simulink library "ammclib_bam_s32k11x"  (Simulink 9.0)
settings: Solver=ode45  StartTime=0.0  StopTime=10.0  RelTol=1e-3
undefined symbols (not defined in the file): f16A1, f16A2, f16B0, f16B1, f16B2, f16C1, f16CC1, f16CC1sc, f16CC1sc_D, f16CC1sc_Q, f16CC1scD, f16CC1scQ, f16CC2, f16CC2sc, f16CC2sc_D, f16CC2sc_Q, f16CC2scD, f16CC2scQ, f16DerivGain, f16EGain, f16FiltCoef, f16HystOff, f16HystOn, f16IGain, f16IntegGain, f16IntegGainFW, f16IntegGainQ, f16Kd, f16Kq, f16Limit, f16LowerLim, f16LowerLimit_D, f16LowerLimit_Q, f16ModIndex, f16OutValOff, f16OutValOn, f16PropGain, f16PropGainFW, f16PropGainQ, f16RampDown, f16RampUp, f16UGain, f16UpperLim, f16UpperLimit, f16UpperLimit_D, f16UpperLimit_Q, f16WIGain, f32A1, f32A2, f32B0, f32B1, f32B2, f32C1, f32CC1, f32CC1sc, f32CC1sc_D, f32CC1sc_Q, f32CC1scD, f32CC1scQ, f32CC2 ... (+71)
(part 3 of 7)

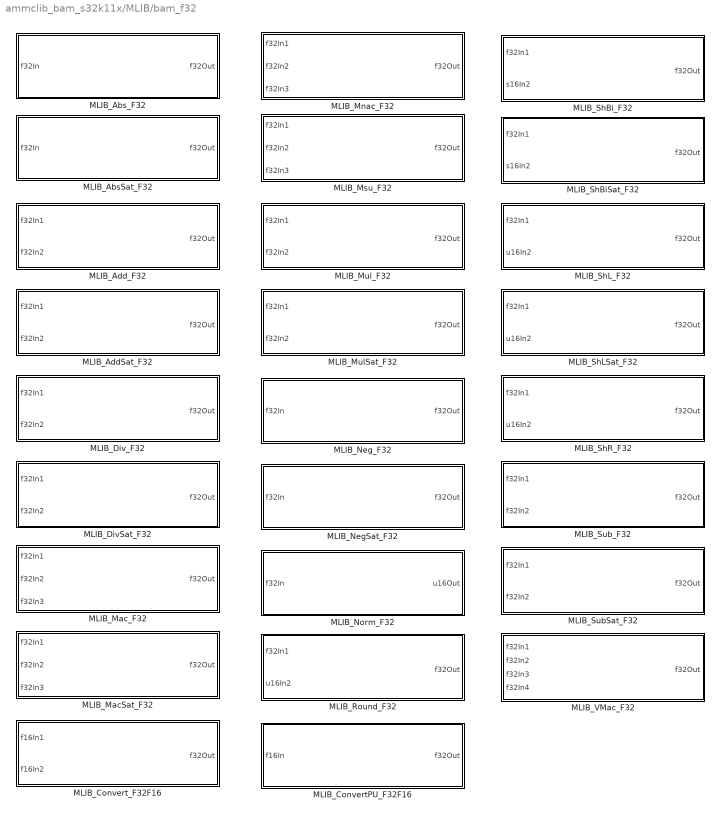
== system ammclib_bam_s32k11x/MLIB/bam_f32 ==
  MLIB_AbsSat_F32 : Subsystem  mask(MLIB_AbsSat_F32){}
      mask help: Bit accurate model for absolute value of input value. The output is saturated if necessary. All parameters as well as input and output are 32bit integers.
      mask init:
      | pos = get_param(gcb, 'Position');width = pos(3) - pos(1); height = pos(4) - pos(2);tX=width/2;tY=height*0.9;
      mask Help: web(fullfile(mbd_s32k_mc_block_help('s32k11x'), 'S32K11XMCLUG.pdf'), '-browser')
      mask Display: color('black');port_label('input',1,'f32In');port_label('output',1,'f32Out');color('black');disp('MLIB_AbsSat_F32');color('blue');text(tX,tY, 'BAM', 'horizontalAlignment', 'center');
  MLIB_Abs_F32 : Subsystem  mask(MLIB_Abs_F32){}
      mask help: Bit accurate model for absolute value of input value. All parameters as well as input and output are 32bit integers.
      mask init:
      | pos = get_param(gcb, 'Position');width = pos(3) - pos(1); height = pos(4) - pos(2);tX=width/2;tY=height*0.9;
      mask Help: web(fullfile(mbd_s32k_mc_block_help('s32k11x'), 'S32K11XMCLUG.pdf'), '-browser')
      mask Display: color('black');port_label('input',1,'f32In');port_label('output',1,'f32Out');color('black');disp('MLIB_Abs_F32');color('blue');text(tX,tY, 'BAM', 'horizontalAlignment', 'center');
  MLIB_AddSat_F32 : Subsystem  mask(MLIB_AddSat_F32){}
      mask help: Bit accurate model of saturated sum of two input values. All parameters as well as input and output are 32bit integers.
      mask init:
      | pos = get_param(gcb, 'Position');width = pos(3) - pos(1); height = pos(4) - pos(2);tX=width/2;tY=height*0.9;
      mask Help: web(fullfile(mbd_s32k_mc_block_help('s32k11x'), 'S32K11XMCLUG.pdf'), '-browser')
      mask Display: color('black');port_label('input',1,'f32In1');port_label('input',2,'f32In2');port_label('output',1,'f32Out');color('black');disp('MLIB_AddSat_F32');color('blue');text(tX,tY, 'BAM', 'horizontalAlignment', 'center');
  MLIB_Add_F32 : Subsystem  mask(MLIB_Add_F32){}
      mask help: Bit accurate model of sum of two input values. All parameters as well as input and output are 32bit integers.
      mask init:
      | pos = get_param(gcb, 'Position');width = pos(3) - pos(1); height = pos(4) - pos(2);tX=width/2;tY=height*0.9;
      mask Help: web(fullfile(mbd_s32k_mc_block_help('s32k11x'), 'S32K11XMCLUG.pdf'), '-browser')
      mask Display: color('black');port_label('input',1,'f32In1');port_label('input',2,'f32In2');port_label('output',1,'f32Out');color('black');disp('MLIB_Add_F32');color('blue');text(tX,tY, 'BAM', 'horizontalAlignment', 'center');
  MLIB_ConvertPU_F32F16 : Subsystem  mask(MLIB_ConvertPU_F32){}
      mask help: Bit accurate model for conversion value of input value. Input parameter is considered as 16-bit integer and output value is considered as 32-bit integer value.
      mask init:
      | pos = get_param(gcb, 'Position');width = pos(3) - pos(1); height = pos(4) - pos(2);tX=width/2;tY=height*0.9;
      mask Help: web(fullfile(mbd_s32k_mc_block_help('s32k11x'), 'S32K11XMCLUG.pdf'), '-browser')
      mask Display: color('black');port_label('input',1,'f16In');port_label('output',1,'f32Out');color('black');disp('MLIB_ConvertPU_F32F16');color('blue');text(tX,tY, 'BAM', 'horizontalAlignment', 'center');
  MLIB_Convert_F32F16 : Subsystem  mask(MLIB_Convert_F32F16){}
      mask help: Bit accurate model for conversion value of input value. Input parameter is considered as 16-bit integer and output value is considered as 32-bit integer value.
      mask init:
      | pos = get_param(gcb, 'Position');width = pos(3) - pos(1); height = pos(4) - pos(2);tX=width/2;tY=height*0.9;
      mask Help: web(fullfile(mbd_s32k_mc_block_help('s32k11x'), 'S32K11XMCLUG.pdf'), '-browser')
      mask Display: color('black');port_label('input',1,'f16In1');port_label('input',2,'f16In2');port_label('output',1,'f32Out');color('black');disp('MLIB_Convert_F32F16');color('blue');text(tX,tY, 'BAM', 'horizontalAlignment', 'center');
  MLIB_DivSat_F32 : Subsystem  mask(MLIB_DivSat_F32){}
      mask help: Bit accurate model of multiplication of two input values. All parameters as well as input and output are 32bit integers.
      mask init:
      | pos = get_param(gcb, 'Position');width = pos(3) - pos(1); height = pos(4) - pos(2);tX=width/2;tY=height*0.9;
      mask Help: web(fullfile(mbd_s32k_mc_block_help('s32k11x'), 'S32K11XMCLUG.pdf'), '-browser')
      mask Display: color('black');port_label('input',1,'f32In1');port_label('input',2,'f32In2');port_label('output',1,'f32Out');color('black');disp('MLIB_DivSat_F32');color('blue');text(tX,tY, 'BAM', 'horizontalAlignment', 'center');
  MLIB_Div_F32 : Subsystem  mask(MLIB_Div_F32){}
      mask help: Bit accurate model of multiplication of two input values. All parameters as well as input and output are 32bit integers.
      mask init:
      | pos = get_param(gcb, 'Position');width = pos(3) - pos(1); height = pos(4) - pos(2);tX=width/2;tY=height*0.9;
      mask Help: web(fullfile(mbd_s32k_mc_block_help('s32k11x'), 'S32K11XMCLUG.pdf'), '-browser')
      mask Display: color('black');port_label('input',1,'f32In1');port_label('input',2,'f32In2');port_label('output',1,'f32Out');color('black');disp('MLIB_Div_F32');color('blue');text(tX,tY, 'BAM', 'horizontalAlignment', 'center');
  MLIB_MacSat_F32 : Subsystem  mask(MLIB_MacSat_F32){}
      mask help: Bit accurate model of saturated multiply-accumulate of input values, saturated if necessary. All parameters as well as input and output are 32bit integers.
      mask init:
      | pos = get_param(gcb, 'Position');width = pos(3) - pos(1); height = pos(4) - pos(2);tX=width/2;tY=height*0.9;
      mask Help: web(fullfile(mbd_s32k_mc_block_help('s32k11x'), 'S32K11XMCLUG.pdf'), '-browser')
      mask Display: color('black');port_label('input',1,'f32In1');port_label('input',2,'f32In2');port_label('input',3,'f32In3');port_label('output',1,'f32Out');color('black');disp('MLIB_MacSat_F32');color('blue');text(tX,tY, 'BAM', 'horizontalAlignment', 'center');
  MLIB_Mac_F32 : Subsystem  mask(MLIB_Mac_F32){}
      mask help: Bit accurate model of multiply accumulate function. All parameters as well as input and output are 32bit integers.
      mask init:
      | pos = get_param(gcb, 'Position');width = pos(3) - pos(1); height = pos(4) - pos(2);tX=width/2;tY=height*0.9;
      mask Help: web(fullfile(mbd_s32k_mc_block_help('s32k11x'), 'S32K11XMCLUG.pdf'), '-browser')
      mask Display: color('black');port_label('input',1,'f32In1');port_label('input',2,'f32In2');port_label('input',3,'f32In3');port_label('output',1,'f32Out');color('black');disp('MLIB_Mac_F32');color('blue');text(tX,tY, 'BAM', 'horizontalAlignment', 'center');
  MLIB_Mnac_F32 : Subsystem  mask(MLIB_Mnac_F32){}
      mask help: Bit accurate model of multiply-negative-accumulate function. All parameters as well as input and output are 32bit integers.
      mask init:
      | pos = get_param(gcb, 'Position');width = pos(3) - pos(1); height = pos(4) - pos(2);tX=width/2;tY=height*0.9;
      mask Help: web(fullfile(mbd_s32k_mc_block_help('s32k11x'), 'S32K11XMCLUG.pdf'), '-browser')
      mask Display: color('black');port_label('input',1,'f32In1');port_label('input',2,'f32In2');port_label('input',3,'f32In3');port_label('output',1,'f32Out');color('black');disp('MLIB_Mnac_F32');color('blue');text(tX,tY, 'BAM', 'horizontalAlignment', 'center');
  MLIB_Msu_F32 : Subsystem  mask(MLIB_Msu_F32){}
      mask help: Bit accurate model of multiply-subtract-from function. All parameters as well as input and output are 32bit integers.
      mask init:
      | pos = get_param(gcb, 'Position');width = pos(3) - pos(1); height = pos(4) - pos(2);tX=width/2;tY=height*0.9;
      mask Help: web(fullfile(mbd_s32k_mc_block_help('s32k11x'), 'S32K11XMCLUG.pdf'), '-browser')
      mask Display: color('black');port_label('input',1,'f32In1');port_label('input',2,'f32In2');port_label('input',3,'f32In3');port_label('output',1,'f32Out');color('black');disp('MLIB_Msu_F32');color('blue');text(tX,tY, 'BAM', 'horizontalAlignment', 'center');
  MLIB_MulSat_F32 : Subsystem  mask(MLIB_MulSat_F32){}
      mask help: Bit accurate model of saturated multiplication of two input values. All parameters as well as input and output are 32bit integers.
      mask init:
      | pos = get_param(gcb, 'Position');width = pos(3) - pos(1); height = pos(4) - pos(2);tX=width/2;tY=height*0.9;
      mask Help: web(fullfile(mbd_s32k_mc_block_help('s32k11x'), 'S32K11XMCLUG.pdf'), '-browser')
      mask Display: color('black');port_label('input',1,'f32In1');port_label('input',2,'f32In2');port_label('output',1,'f32Out');color('black');disp('MLIB_MulSat_F32');color('blue');text(tX,tY, 'BAM', 'horizontalAlignment', 'center');
  MLIB_Mul_F32 : Subsystem  mask(MLIB_Mul_F32){}
      mask help: Bit accurate model of multiplication of two input values. All parameters as well as input and output are 32bit integers.
      mask init:
      | pos = get_param(gcb, 'Position');width = pos(3) - pos(1); height = pos(4) - pos(2);tX=width/2;tY=height*0.9;
      mask Help: web(fullfile(mbd_s32k_mc_block_help('s32k11x'), 'S32K11XMCLUG.pdf'), '-browser')
      mask Display: color('black');port_label('input',1,'f32In1');port_label('input',2,'f32In2');port_label('output',1,'f32Out');color('black');disp('MLIB_Mul_F32');color('blue');text(tX,tY, 'BAM', 'horizontalAlignment', 'center');
  MLIB_NegSat_F32 : Subsystem  mask(MLIB_NegSat_F32){}
      mask help: Bit accurate model for negative value of input value. The output is saturated if necessary. All parameters as well as input and output are 32bit integers.
      mask init:
      | pos = get_param(gcb, 'Position');width = pos(3) - pos(1); height = pos(4) - pos(2);tX=width/2;tY=height*0.9;
      mask Help: web(fullfile(mbd_s32k_mc_block_help('s32k11x'), 'S32K11XMCLUG.pdf'), '-browser')
      mask Display: color('black');port_label('input',1,'f32In');port_label('output',1,'f32Out');color('black');disp('MLIB_NegSat_F32');color('blue');text(tX,tY, 'BAM', 'horizontalAlignment', 'center');
  MLIB_Neg_F32 : Subsystem  mask(MLIB_Neg_F32){}
      mask help: Bit accurate model for negative value of input value. All parameters as well as input and output are 32bit integers.
      mask init:
      | pos = get_param(gcb, 'Position');width = pos(3) - pos(1); height = pos(4) - pos(2);tX=width/2;tY=height*0.9;
      mask Help: web(fullfile(mbd_s32k_mc_block_help('s32k11x'), 'S32K11XMCLUG.pdf'), '-browser')
      mask Display: color('black');port_label('input',1,'f32In');port_label('output',1,'f32Out');color('black');disp('MLIB_Neg_F32');color('blue');text(tX,tY, 'BAM', 'horizontalAlignment', 'center');
  MLIB_Norm_F32 : Subsystem  mask(MLIB_Norm_F32){}
      mask help: Bit accurate model of the normalization function. The function counts the number of left shift needed for normalization of the input fractional value.
      mask init:
      | pos = get_param(gcb, 'Position');width = pos(3) - pos(1); height = pos(4) - pos(2);tX=width/2;tY=height*0.9;
      mask Help: web(fullfile(mbd_s32k_mc_block_help('s32k11x'), 'S32K11XMCLUG.pdf'), '-browser')
      mask Display: color('black');port_label('input',1,'f32In');port_label('output',1,'u16Out');color('black');disp('MLIB_Norm_F32');color('blue');text(tX,tY, 'BAM', 'horizontalAlignment', 'center');
  MLIB_Round_F32 : Subsystem  mask(MLIB_Round_F32){}
      mask help: Bit accurate model of the fuction rounds the first input value for number of digits defined by second parameter and saturate automaticaly. All parameters as well as input and output are 32bit integers.
      mask init:
      | pos = get_param(gcb, 'Position');width = pos(3) - pos(1); height = pos(4) - pos(2);tX=width/2;tY=height*0.9;
      mask Help: web(fullfile(mbd_s32k_mc_block_help('s32k11x'), 'S32K11XMCLUG.pdf'), '-browser')
      mask Display: color('black');port_label('input',1,'f32In1');port_label('input',2,'u16In2');port_label('output',1,'f32Out');color('black');disp('MLIB_Round_F32');color('blue');text(tX,tY, 'BAM', 'horizontalAlignment', 'center');
  MLIB_ShBiSat_F32 : Subsystem  mask(MLIB_ShBiSat_F32){}
      mask help: Bit accurate model of the fuction shifts the first parameter to left or right by number defined by second parameter and saturate if necessary. If the sign of second parameter is negative, shift to right. All parameters as well as input and output are 32bit integers.
      mask init:
      | pos = get_param(gcb, 'Position');width = pos(3) - pos(1); height = pos(4) - pos(2);tX=width/2;tY=height*0.9;
      mask Help: web(fullfile(mbd_s32k_mc_block_help('s32k11x'), 'S32K11XMCLUG.pdf'), '-browser')
      mask Display: color('black');port_label('input',1,'f32In1');port_label('input',2,'s16In2');port_label('output',1,'f32Out');color('black');disp('MLIB_ShBiSat_F32');color('blue');text(tX,tY, 'BAM', 'horizontalAlignment', 'center');
  MLIB_ShBi_F32 : Subsystem  mask(MLIB_ShBi_F32){}
      mask help: Bit accurate model of the fuction shifts the first parameter to left or right by number defined by second parameter. If the sign of second parameter is negative, shift to right. All parameters as well as input and output are 16bit integers.
      mask init:
      | pos = get_param(gcb, 'Position');width = pos(3) - pos(1); height = pos(4) - pos(2);tX=width/2;tY=height*0.9;
      mask Help: web(fullfile(mbd_s32k_mc_block_help('s32k11x'), 'S32K11XMCLUG.pdf'), '-browser')
      mask Display: color('black');port_label('input',1,'f32In1');port_label('input',2,'s16In2');port_label('output',1,'f32Out');color('black');disp('MLIB_ShBi_F32');color('blue');text(tX,tY, 'BAM', 'horizontalAlignment', 'center');
  MLIB_ShLSat_F32 : Subsystem  mask(MLIB_ShLSat_F32){}
      mask help: Bit accurate model of the fuction shifts the first parameter to left by number defined by second parameter and saturate if necessary. All parameters as well as input and output are 32bit integers.
      mask init:
      | pos = get_param(gcb, 'Position');width = pos(3) - pos(1); height = pos(4) - pos(2);tX=width/2;tY=height*0.9;
      mask Help: web(fullfile(mbd_s32k_mc_block_help('s32k11x'), 'S32K11XMCLUG.pdf'), '-browser')
      mask Display: color('black');port_label('input',1,'f32In1');port_label('input',2,'u16In2');port_label('output',1,'f32Out');color('black');disp('MLIB_ShLSat_F32');color('blue');text(tX,tY, 'BAM', 'horizontalAlignment', 'center');
  MLIB_ShL_F32 : Subsystem  mask(MLIB_ShL_F32){}
      mask help: Bit accurate model of the fuction shifts the first parameter to left by number defined by second parameter. All parameters as well as input and output are 32bit integers.
      mask init:
      | pos = get_param(gcb, 'Position');width = pos(3) - pos(1); height = pos(4) - pos(2);tX=width/2;tY=height*0.9;
      mask Help: web(fullfile(mbd_s32k_mc_block_help('s32k11x'), 'S32K11XMCLUG.pdf'), '-browser')
      mask Display: color('black');port_label('input',1,'f32In1');port_label('input',2,'u16In2');port_label('output',1,'f32Out');color('black');disp('MLIB_ShL_F32');color('blue');text(tX,tY, 'BAM', 'horizontalAlignment', 'center');
  MLIB_ShR_F32 : Subsystem  mask(MLIB_ShR_F32){}
      mask help: Bit accurate model of the fuction shifts the first parameter to right by number defined by second parameter. All parameters as well as input and output are 32bit integers.
      mask init:
      | pos = get_param(gcb, 'Position');width = pos(3) - pos(1); height = pos(4) - pos(2);tX=width/2;tY=height*0.9;
      mask Help: web(fullfile(mbd_s32k_mc_block_help('s32k11x'), 'S32K11XMCLUG.pdf'), '-browser')
      mask Display: color('black');port_label('input',1,'f32In1');port_label('input',2,'u16In2');port_label('output',1,'f32Out');color('black');disp('MLIB_ShR_F32');color('blue');text(tX,tY, 'BAM', 'horizontalAlignment', 'center');
  MLIB_SubSat_F32 : Subsystem  mask(MLIB_SubSat_F32){}
      mask help: Bit accurate model of saturated subtraction of two input values. All parameters as well as input and output are 32bit integers.
      mask init:
      | pos = get_param(gcb, 'Position');width = pos(3) - pos(1); height = pos(4) - pos(2);tX=width/2;tY=height*0.9;
      mask Help: web(fullfile(mbd_s32k_mc_block_help('s32k11x'), 'S32K11XMCLUG.pdf'), '-browser')
      mask Display: color('black');port_label('input',1,'f32In1');port_label('input',2,'f32In2');port_label('output',1,'f32Out');color('black');disp('MLIB_SubSat_F32');color('blue');text(tX,tY, 'BAM', 'horizontalAlignment', 'center');
  MLIB_Sub_F32 : Subsystem  mask(MLIB_Sub_F32){}
      mask help: Bit accurate model of subtract of two input values. All parameters as well as input and output are 32bit integers.
      mask init:
      | pos = get_param(gcb, 'Position');width = pos(3) - pos(1); height = pos(4) - pos(2);tX=width/2;tY=height*0.9;
      mask Help: web(fullfile(mbd_s32k_mc_block_help('s32k11x'), 'S32K11XMCLUG.pdf'), '-browser')
      mask Display: color('black');port_label('input',1,'f32In1');port_label('input',2,'f32In2');port_label('output',1,'f32Out');color('black');disp('MLIB_Sub_F32');color('blue');text(tX,tY, 'BAM', 'horizontalAlignment', 'center');
  MLIB_VMac_F32 : Subsystem  mask(MLIB_VMac_F32){}
      mask help: Bit accurate model of vector multiply accumulate function. All parameters as well as input and output are 32-bit integers.
      mask init:
      | pos = get_param(gcb, 'Position');width = pos(3) - pos(1); height = pos(4) - pos(2);tX=width/2;tY=height*0.9;
      mask Help: web(fullfile(mbd_s32k_mc_block_help('s32k11x'), 'S32K11XMCLUG.pdf'), '-browser')
      mask Display: color('black');port_label('input',1,'f32In1');port_label('input',2,'f32In2');port_label('input',3,'f32In3');port_label('input',4,'f32In4');port_label('output',1,'f32Out');color('black');disp('MLIB_VMac_F32');color('blue');text(tX,tY, 'BAM', 'horizontalAlignment', 'center');

== system ammclib_bam_s32k11x/MLIB/bam_f32f16f16 ==
  MLIB_MacSat_F32F16F16 : Subsystem  mask(MLIB_MacSat_F32F16F16){}
      mask help: Bit accurate model of saturated multiply-accumulate of input values, saturated if necessary. All input parameters are 16bit integers, output value is 32-bit integer.
      mask init:
      | pos = get_param(gcb, 'Position');width = pos(3) - pos(1); height = pos(4) - pos(2);tX=width/2;tY=height*0.9;
      mask Help: web(fullfile(mbd_s32k_mc_block_help('s32k11x'), 'S32K11XMCLUG.pdf'), '-browser')
      mask Display: color('black');port_label('input',1,'f32In1');port_label('input',2,'f16In2');port_label('input',3,'f16In3');port_label('output',1,'f32Out');color('black');disp('MLIB_MacSat_F32F16F16');color('blue');text(tX,tY, 'BAM', 'horizontalAlignment', 'center');
  MLIB_Mac_F32F16F16 : Subsystem  mask(MLIB_Mac_F32F16F16){}
      mask help: Bit accurate model of multiply accumulate function. First input parameters as well as output are 32bit integers. Second and third parameters are 16-bit integers.
      mask init:
      | pos = get_param(gcb, 'Position');width = pos(3) - pos(1); height = pos(4) - pos(2);tX=width/2;tY=height*0.9;
      mask Help: web(fullfile(mbd_s32k_mc_block_help('s32k11x'), 'S32K11XMCLUG.pdf'), '-browser')
      mask Display: color('black');port_label('input',1,'f32In1');port_label('input',2,'f16In2');port_label('input',3,'f16In3');port_label('output',1,'f32Out');color('black');disp('MLIB_Mac_F32F16F16');color('blue');text(tX,tY, 'BAM', 'horizontalAlignment', 'center');
  MLIB_Mnac_F32F16F16 : Subsystem  mask(MLIB_Mnac_F32F16F16){}
      mask help: Bit accurate model of multiply-negative-accumulate function. First input parameters as well as output are 32bit integers. Second and third parameters are 16-bit integers.
      mask init:
      | pos = get_param(gcb, 'Position');width = pos(3) - pos(1); height = pos(4) - pos(2);tX=width/2;tY=height*0.9;
      mask Help: web(fullfile(mbd_s32k_mc_block_help('s32k11x'), 'S32K11XMCLUG.pdf'), '-browser')
      mask Display: color('black');port_label('input',1,'f32In1');port_label('input',2,'f16In2');port_label('input',3,'f16In3');port_label('output',1,'f32Out');color('black');disp('MLIB_Mnac_F32F16F16');color('blue');text(tX,tY, 'BAM', 'horizontalAlignment', 'center');
  MLIB_Msu_F32F16F16 : Subsystem  mask(MLIB_Msu_F32F16F16){}
      mask help: Bit accurate model of multiply-subtract-from function. First input parameter as well as output are 32bit integers. Second and third parameters are 16-bit integers.
      mask init:
      | pos = get_param(gcb, 'Position');width = pos(3) - pos(1); height = pos(4) - pos(2);tX=width/2;tY=height*0.9;
      mask Help: web(fullfile(mbd_s32k_mc_block_help('s32k11x'), 'S32K11XMCLUG.pdf'), '-browser')
      mask Display: color('black');port_label('input',1,'f32In1');port_label('input',2,'f16In2');port_label('input',3,'f16In3');port_label('output',1,'f32Out');color('black');disp('MLIB_Msu_F32F16F16');color('blue');text(tX,tY, 'BAM', 'horizontalAlignment', 'center');
  MLIB_MulSat_F32F16F16 : Subsystem  mask(MLIB_MulSat_F32F16F16){}
      mask help: Bit accurate model of saturated multiplication of two input values. All input parameters are 16bit integers, output value is 32-bit integer.
      mask init:
      | pos = get_param(gcb, 'Position');width = pos(3) - pos(1); height = pos(4) - pos(2);tX=width/2;tY=height*0.9;
      mask Help: web(fullfile(mbd_s32k_mc_block_help('s32k11x'), 'S32K11XMCLUG.pdf'), '-browser')
      mask Display: color('black');port_label('input',1,'f16In1');port_label('input',2,'f16In2');port_label('output',1,'f32Out');color('black');disp('MLIB_MulSat_F32F16F16');color('blue');text(tX,tY, 'BAM', 'horizontalAlignment', 'center');
  MLIB_Mul_F32F16F16 : Subsystem  mask(MLIB_Mul_F32F16F16){}
      mask help: Bit accurate model of multiplication of two input values. Both input parameters are 16bit integers and output value is 32-bit integer.
      mask init:
      | pos = get_param(gcb, 'Position');width = pos(3) - pos(1); height = pos(4) - pos(2);tX=width/2;tY=height*0.9;
      mask Help: web(fullfile(mbd_s32k_mc_block_help('s32k11x'), 'S32K11XMCLUG.pdf'), '-browser')
      mask Display: color('black');port_label('input',1,'f16In1');port_label('input',2,'f16In2');port_label('output',1,'f32Out');color('black');disp('MLIB_Mul_F32F16F16');color('blue');text(tX,tY, 'BAM', 'horizontalAlignment', 'center');
  MLIB_VMac_F32F16F16 : Subsystem  mask(MLIB_VMac_F32F16F16){}
      mask help: Bit accurate model of vector multiply accumulate function. The input parameters are 16-bit integers, the output value is 32-bit integer.
      mask init:
      | pos = get_param(gcb, 'Position');width = pos(3) - pos(1); height = pos(4) - pos(2);tX=width/2;tY=height*0.9;
      mask Help: web(fullfile(mbd_s32k_mc_block_help('s32k11x'), 'S32K11XMCLUG.pdf'), '-browser')
      mask Display: color('black');port_label('input',1,'f16In1');port_label('input',2,'f16In2');port_label('input',3,'f16In3');port_label('input',4,'f16In4');port_label('output',1,'f32Out');color('black');disp('MLIB_VMac_F32F16F16');color('blue');text(tX,tY, 'BAM', 'horizontalAlignment', 'center');

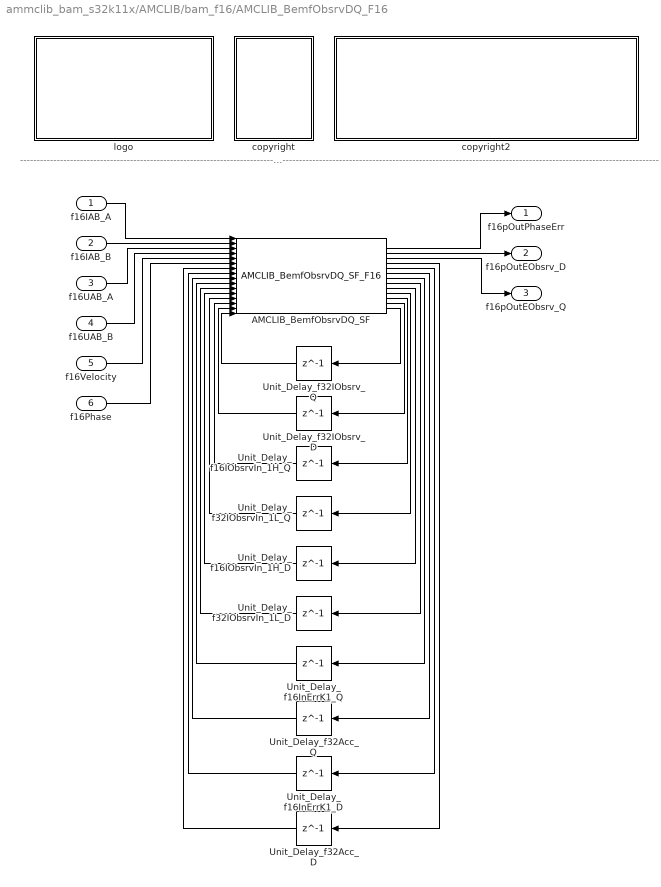
== system ammclib_bam_s32k11x/AMCLIB/bam_f16/AMCLIB_BemfObsrvDQ_F16 ==
  note: ---------------------------------------------------------------------------------------------------------------------------------------------------------------------------------------------------
  f16IAB_A : Inport
  f16IAB_B : Inport  Port=2
  f16UAB_A : Inport  Port=3
  f16UAB_B : Inport  Port=4
  f16Velocity : Inport  Port=5
  f16Phase : Inport  Port=6
  AMCLIB_BemfObsrvDQ_SF : S-Function  FunctionName=AMCLIB_BemfObsrvDQ_SF_F16  Parameters=f16IGain,f16UGain,f16WIGain,f16EGain,s16Shift,f16CC1sc_D,f16CC1sc_Q,f16CC2sc_D,f16CC2sc_Q,f16UpperLimit_D,f16UpperLimit_Q,f16LowerLimit_D,f16LowerLimit_Q,u16NShift  SFunctionDeploymentMode=off  EnableBusSupport=off
  Unit_Delay_f16IObsrvIn_1H_D : Delay  DelayLength=1  InitialCondition=0
  Unit_Delay_f16IObsrvIn_1H_Q : Delay  DelayLength=1  InitialCondition=0
  Unit_Delay_f16InErrK1_D : Delay  DelayLength=1  InitialCondition=0
  Unit_Delay_f16InErrK1_Q : Delay  DelayLength=1  InitialCondition=0
  Unit_Delay_f32Acc_D : Delay  DelayLength=1  InitialCondition=0
  Unit_Delay_f32Acc_Q : Delay  DelayLength=1  InitialCondition=0
  Unit_Delay_f32IObsrvIn_1L_D : Delay  DelayLength=1  InitialCondition=0
  Unit_Delay_f32IObsrvIn_1L_Q : Delay  DelayLength=1  InitialCondition=0
  Unit_Delay_f32IObsrv_D : Delay  DelayLength=1  InitialCondition=0
  Unit_Delay_f32IObsrv_Q : Delay  DelayLength=1  InitialCondition=0
  copyright : Subsystem
      mask Display: text(10,90,'FILE:');text(10,75,'DESRIPTION:');text(10,60,'COPYRIGHT:');text(10,45,'VERSION:');text(10,30,'DATE:')
  copyright2 : Subsystem
      mask Display: text(10,90,'AMCLIB_BemfObsrvDQ_BAM_F16.mdl');text(10,75,'PMSM back-EMF observer DQ.');text(10,60,'NXP');text(10,45,'1.0');text(10,30,'26-Oct-2016');
  logo : Subsystem
      mask Display: image(imread('logo.jpg'))
  f16pOutPhaseErr : Outport
  f16pOutEObsrv_D : Outport  Port=2
  f16pOutEObsrv_Q : Outport  Port=3
  wires:
  f16IAB_A/1 -> AMCLIB_BemfObsrvDQ_SF/1
  f16IAB_B/1 -> AMCLIB_BemfObsrvDQ_SF/2
  f16UAB_A/1 -> AMCLIB_BemfObsrvDQ_SF/3
  f16UAB_B/1 -> AMCLIB_BemfObsrvDQ_SF/4
  f16Velocity/1 -> AMCLIB_BemfObsrvDQ_SF/5
  f16Phase/1 -> AMCLIB_BemfObsrvDQ_SF/6
  AMCLIB_BemfObsrvDQ_SF/1 -> f16pOutPhaseErr/1
  AMCLIB_BemfObsrvDQ_SF/2 -> f16pOutEObsrv_D/1
  AMCLIB_BemfObsrvDQ_SF/3 -> f16pOutEObsrv_Q/1
  Unit_Delay_f32IObsrv_Q/1 -> AMCLIB_BemfObsrvDQ_SF/16
  Unit_Delay_f32IObsrv_D/1 -> AMCLIB_BemfObsrvDQ_SF/15
  Unit_Delay_f16IObsrvIn_1H_Q/1 -> AMCLIB_BemfObsrvDQ_SF/14
  AMCLIB_BemfObsrvDQ_SF/13 -> Unit_Delay_f32IObsrv_Q/1
  AMCLIB_BemfObsrvDQ_SF/12 -> Unit_Delay_f32IObsrv_D/1
  AMCLIB_BemfObsrvDQ_SF/11 -> Unit_Delay_f16IObsrvIn_1H_Q/1
  Unit_Delay_f32IObsrvIn_1L_Q/1 -> AMCLIB_BemfObsrvDQ_SF/13
  AMCLIB_BemfObsrvDQ_SF/10 -> Unit_Delay_f32IObsrvIn_1L_Q/1
  Unit_Delay_f16IObsrvIn_1H_D/1 -> AMCLIB_BemfObsrvDQ_SF/12
  AMCLIB_BemfObsrvDQ_SF/9 -> Unit_Delay_f16IObsrvIn_1H_D/1
  Unit_Delay_f32IObsrvIn_1L_D/1 -> AMCLIB_BemfObsrvDQ_SF/11
  AMCLIB_BemfObsrvDQ_SF/8 -> Unit_Delay_f32IObsrvIn_1L_D/1
  Unit_Delay_f16InErrK1_Q/1 -> AMCLIB_BemfObsrvDQ_SF/10
  AMCLIB_BemfObsrvDQ_SF/7 -> Unit_Delay_f16InErrK1_Q/1
  Unit_Delay_f32Acc_Q/1 -> AMCLIB_BemfObsrvDQ_SF/9
  AMCLIB_BemfObsrvDQ_SF/6 -> Unit_Delay_f32Acc_Q/1
  AMCLIB_BemfObsrvDQ_SF/5 -> Unit_Delay_f16InErrK1_D/1
  Unit_Delay_f16InErrK1_D/1 -> AMCLIB_BemfObsrvDQ_SF/8
  Unit_Delay_f32Acc_D/1 -> AMCLIB_BemfObsrvDQ_SF/7
  AMCLIB_BemfObsrvDQ_SF/4 -> Unit_Delay_f32Acc_D/1

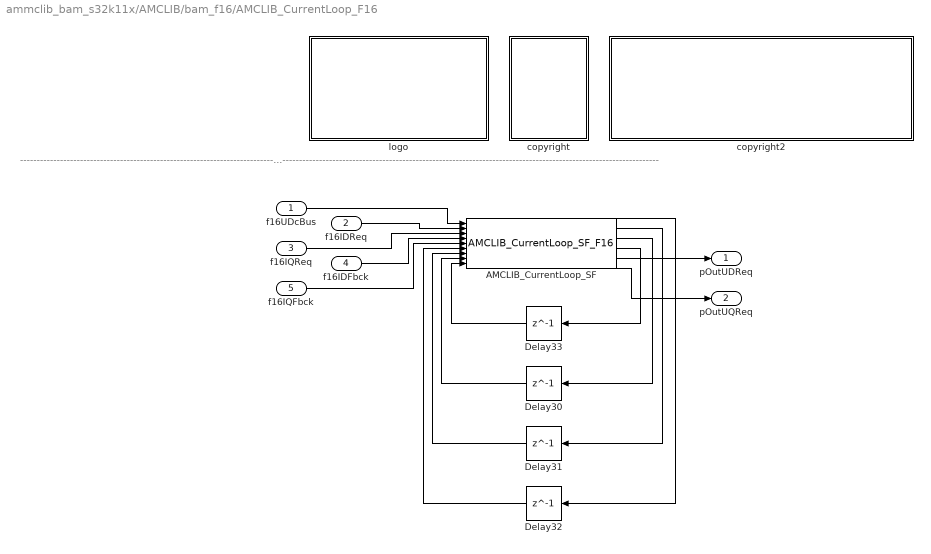
== system ammclib_bam_s32k11x/AMCLIB/bam_f16/AMCLIB_CurrentLoop_F16 ==
  note: ---------------------------------------------------------------------------------------------------------------------------------------------------------------------------------------------------
  f16UDcBus : Inport
  f16IDReq : Inport  Port=2
  f16IQReq : Inport  Port=3
  f16IDFbck : Inport  Port=4
  f16IQFbck : Inport  Port=5
  AMCLIB_CurrentLoop_SF : S-Function  FunctionName=AMCLIB_CurrentLoop_SF_F16  Parameters=f16CC1scD,f16CC2scD,u16NShiftD,f16CC1scQ,f16CC2scQ,u16NShiftQ  SFunctionDeploymentMode=off  EnableBusSupport=off
  Delay{30..33} (4 alike) : Delay  DelayLength=1  InitialCondition=0
  copyright : Subsystem
      mask Display: text(10,90,'FILE:');text(10,75,'DESRIPTION:');text(10,60,'COPYRIGHT:');text(10,45,'VERSION:');text(10,30,'DATE:')
  copyright2 : Subsystem
      mask Display: text(10,90,'AMCLIB_CurrentLoop_BAM_F16.mdl');text(10,75,'PMSM Current Loop.');text(10,60,'NXP');text(10,45,'1.0');text(10,30,'25-Oct-2017');
  logo : Subsystem
      mask Display: image(imread('logo.jpg'))
  pOutUDReq : Outport
  pOutUQReq : Outport  Port=2
  wires:
  f16UDcBus/1 -> AMCLIB_CurrentLoop_SF/1
  f16IDReq/1 -> AMCLIB_CurrentLoop_SF/2
  f16IQReq/1 -> AMCLIB_CurrentLoop_SF/3
  f16IDFbck/1 -> AMCLIB_CurrentLoop_SF/4
  f16IQFbck/1 -> AMCLIB_CurrentLoop_SF/5
  Delay32/1 -> AMCLIB_CurrentLoop_SF/6
  Delay31/1 -> AMCLIB_CurrentLoop_SF/7
  Delay30/1 -> AMCLIB_CurrentLoop_SF/8
  Delay33/1 -> AMCLIB_CurrentLoop_SF/9
  AMCLIB_CurrentLoop_SF/1 -> Delay32/1
  AMCLIB_CurrentLoop_SF/2 -> Delay31/1
  AMCLIB_CurrentLoop_SF/3 -> Delay30/1
  AMCLIB_CurrentLoop_SF/4 -> Delay33/1
  AMCLIB_CurrentLoop_SF/5 -> pOutUDReq/1
  AMCLIB_CurrentLoop_SF/6 -> pOutUQReq/1

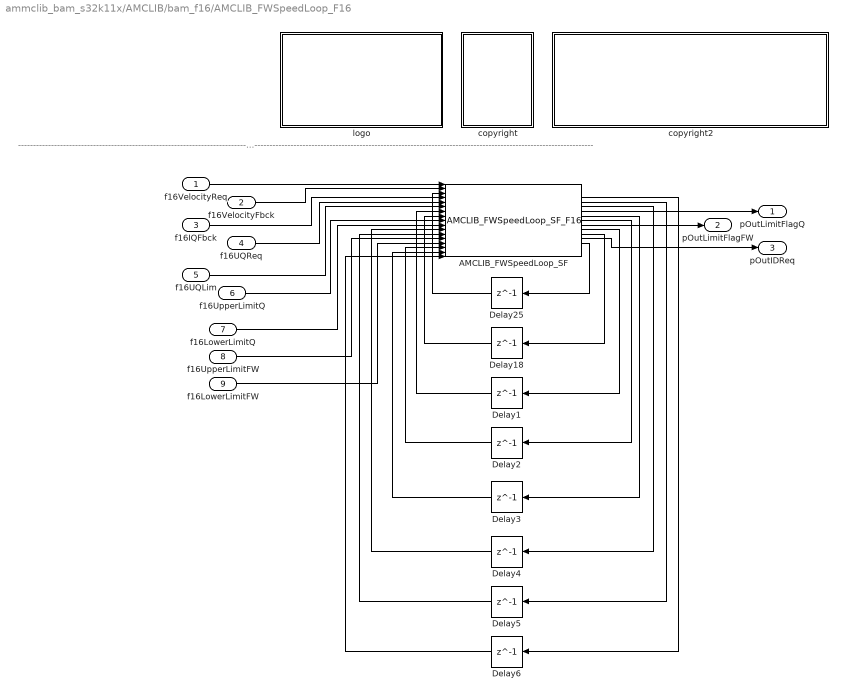
== system ammclib_bam_s32k11x/AMCLIB/bam_f16/AMCLIB_FWSpeedLoop_F16 ==
  note: ---------------------------------------------------------------------------------------------------------------------------------------------------------------------------------------------------
  f16VelocityReq : Inport
  f16VelocityFbck : Inport  Port=2
  f16IQFbck : Inport  Port=3
  f16UQReq : Inport  Port=4
  f16UQLim : Inport  Port=5
  f16UpperLimitQ : Inport  Port=6
  f16LowerLimitQ : Inport  Port=7
  f16UpperLimitFW : Inport  Port=8
  f16LowerLimitFW : Inport  Port=9
  AMCLIB_FWSpeedLoop_SF : S-Function  FunctionName=AMCLIB_FWSpeedLoop_SF_F16  Parameters=u16NSamplesW,u16NSamplesFW,f16PropGainQ,s16PropGainShiftQ,f16IntegGainQ,s16IntegGainShiftQ,f16PropGainFW,s16PropGainShiftFW,f16IntegGainFW,s16IntegGainShiftFW,f32RampUp,f32RampDown  SFunctionDeploymentMode=off  EnableBusSupport=off
  Delay{1..6,18,25} (8 alike) : Delay  DelayLength=1  InitialCondition=0
  copyright : Subsystem
      mask Display: text(10,90,'FILE:');text(10,75,'DESRIPTION:');text(10,60,'COPYRIGHT:');text(10,45,'VERSION:');text(10,30,'DATE:')
  copyright2 : Subsystem
      mask Display: text(10,90,'AMCLIB_FWSpeedLoop_BAM_F16.mdl');text(10,75,'Speed Loop with Field Weakening.');text(10,60,'NXP');text(10,45,'1.0');text(10,30,'28-Aug-2017');
  logo : Subsystem
      mask Display: image(imread('logo.jpg'))
  pOutLimitFlagQ : Outport
  pOutLimitFlagFW : Outport  Port=2
  pOutIDReq : Outport  Port=3
  wires:
  f16VelocityReq/1 -> AMCLIB_FWSpeedLoop_SF/1
  f16VelocityFbck/1 -> AMCLIB_FWSpeedLoop_SF/2
  Delay25/1 -> AMCLIB_FWSpeedLoop_SF/3
  f16IQFbck/1 -> AMCLIB_FWSpeedLoop_SF/4
  f16UQReq/1 -> AMCLIB_FWSpeedLoop_SF/5
  f16UQLim/1 -> AMCLIB_FWSpeedLoop_SF/6
  Delay1/1 -> AMCLIB_FWSpeedLoop_SF/7
  Delay18/1 -> AMCLIB_FWSpeedLoop_SF/8
  f16UpperLimitQ/1 -> AMCLIB_FWSpeedLoop_SF/9
  f16LowerLimitQ/1 -> AMCLIB_FWSpeedLoop_SF/10
  Delay4/1 -> AMCLIB_FWSpeedLoop_SF/11
  Delay5/1 -> AMCLIB_FWSpeedLoop_SF/12
  f16UpperLimitFW/1 -> AMCLIB_FWSpeedLoop_SF/13
  f16LowerLimitFW/1 -> AMCLIB_FWSpeedLoop_SF/14
  Delay2/1 -> AMCLIB_FWSpeedLoop_SF/15
  Delay3/1 -> AMCLIB_FWSpeedLoop_SF/16
  Delay6/1 -> AMCLIB_FWSpeedLoop_SF/17
  AMCLIB_FWSpeedLoop_SF/1 -> Delay6/1
  AMCLIB_FWSpeedLoop_SF/2 -> Delay5/1
  AMCLIB_FWSpeedLoop_SF/3 -> Delay4/1
  AMCLIB_FWSpeedLoop_SF/4 -> pOutLimitFlagQ/1
  AMCLIB_FWSpeedLoop_SF/5 -> Delay3/1
  AMCLIB_FWSpeedLoop_SF/6 -> Delay2/1
  AMCLIB_FWSpeedLoop_SF/7 -> pOutLimitFlagFW/1
  AMCLIB_FWSpeedLoop_SF/8 -> Delay1/1
  AMCLIB_FWSpeedLoop_SF/9 -> Delay18/1
  AMCLIB_FWSpeedLoop_SF/10 -> pOutIDReq/1
  AMCLIB_FWSpeedLoop_SF/11 -> Delay25/1

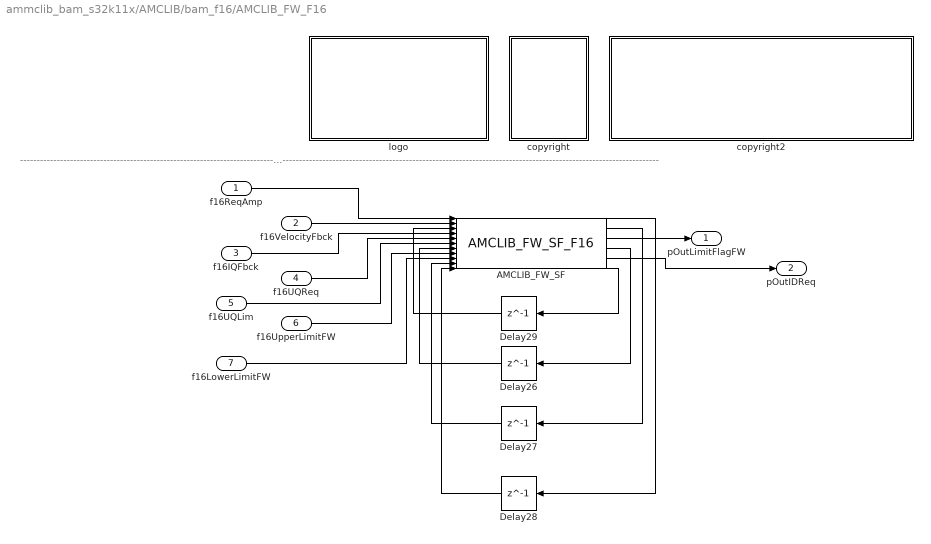
== system ammclib_bam_s32k11x/AMCLIB/bam_f16/AMCLIB_FW_F16 ==
  note: ---------------------------------------------------------------------------------------------------------------------------------------------------------------------------------------------------
  f16ReqAmp : Inport
  f16VelocityFbck : Inport  Port=2
  f16IQFbck : Inport  Port=3
  f16UQReq : Inport  Port=4
  f16UQLim : Inport  Port=5
  f16UpperLimitFW : Inport  Port=6
  f16LowerLimitFW : Inport  Port=7
  AMCLIB_FW_SF : S-Function  FunctionName=AMCLIB_FW_SF_F16  Parameters=u16NSamplesFW,f16PropGainFW,s16PropGainShiftFW,f16IntegGainFW,s16IntegGainShiftFW  SFunctionDeploymentMode=off  EnableBusSupport=off
  Delay{26..29} (4 alike) : Delay  DelayLength=1  InitialCondition=0
  copyright : Subsystem
      mask Display: text(10,90,'FILE:');text(10,75,'DESRIPTION:');text(10,60,'COPYRIGHT:');text(10,45,'VERSION:');text(10,30,'DATE:')
  copyright2 : Subsystem
      mask Display: text(10,90,'AMCLIB_FW_BAM_F16.mdl');text(10,75,'Speed Loop with Field Weakening.');text(10,60,'NXP');text(10,45,'1.0');text(10,30,'28-Aug-2017');
  logo : Subsystem
      mask Display: image(imread('logo.jpg'))
  pOutLimitFlagFW : Outport
  pOutIDReq : Outport  Port=2
  wires:
  f16ReqAmp/1 -> AMCLIB_FW_SF/1
  f16VelocityFbck/1 -> AMCLIB_FW_SF/2
  Delay29/1 -> AMCLIB_FW_SF/3
  f16IQFbck/1 -> AMCLIB_FW_SF/4
  f16UQReq/1 -> AMCLIB_FW_SF/5
  f16UQLim/1 -> AMCLIB_FW_SF/6
  Delay26/1 -> AMCLIB_FW_SF/7
  f16UpperLimitFW/1 -> AMCLIB_FW_SF/8
  f16LowerLimitFW/1 -> AMCLIB_FW_SF/9
  Delay27/1 -> AMCLIB_FW_SF/10
  Delay28/1 -> AMCLIB_FW_SF/11
  AMCLIB_FW_SF/1 -> Delay28/1
  AMCLIB_FW_SF/2 -> Delay27/1
  AMCLIB_FW_SF/3 -> pOutLimitFlagFW/1
  AMCLIB_FW_SF/4 -> Delay26/1
  AMCLIB_FW_SF/5 -> pOutIDReq/1
  AMCLIB_FW_SF/6 -> Delay29/1

== system ammclib_bam_s32k11x/AMCLIB/bam_f16/AMCLIB_SpeedLoop_F16 ==
  note: ---------------------------------------------------------------------------------------------------------------------------------------------------------------------------------------------------
  f16VelocityReq : Inport
  f16VelocityFbck : Inport  Port=2
  f16UpperLimitQ : Inport  Port=3
  f16LowerLimitQ : Inport  Port=4
  AMCLIB_SpeedLoop_SF : S-Function  FunctionName=AMCLIB_SpeedLoop_SF_F16  Parameters=u16NSamplesW,f16PropGainQ,s16PropGainShiftQ,f16IntegGainQ,s16IntegGainShiftQ,f32RampUp,f32RampDown  SFunctionDeploymentMode=off  EnableBusSupport=off
  Delay{1..3,17} (4 alike) : Delay  DelayLength=1  InitialCondition=0
  copyright : Subsystem
      mask Display: text(10,90,'FILE:');text(10,75,'DESRIPTION:');text(10,60,'COPYRIGHT:');text(10,45,'VERSION:');text(10,30,'DATE:')
  copyright2 : Subsystem
      mask Display: text(10,90,'AMCLIB_SpeedLoop_BAM_F16.mdl');text(10,75,'Speed Loop with Field Weakening.');text(10,60,'NXP');text(10,45,'1.0');text(10,30,'28-Aug-2017');
  logo : Subsystem
      mask Display: image(imread('logo.jpg'))
  pOutLimitFlagQ : Outport
  pOutIQReq : Outport  Port=2
  wires:
  f16VelocityReq/1 -> AMCLIB_SpeedLoop_SF/1
  f16VelocityFbck/1 -> AMCLIB_SpeedLoop_SF/2
  Delay17/1 -> AMCLIB_SpeedLoop_SF/3
  f16UpperLimitQ/1 -> AMCLIB_SpeedLoop_SF/4
  f16LowerLimitQ/1 -> AMCLIB_SpeedLoop_SF/5
  Delay1/1 -> AMCLIB_SpeedLoop_SF/6
  Delay2/1 -> AMCLIB_SpeedLoop_SF/7
  Delay3/1 -> AMCLIB_SpeedLoop_SF/8
  AMCLIB_SpeedLoop_SF/1 -> Delay3/1
  AMCLIB_SpeedLoop_SF/2 -> Delay2/1
  AMCLIB_SpeedLoop_SF/3 -> Delay1/1
  AMCLIB_SpeedLoop_SF/4 -> pOutLimitFlagQ/1
  AMCLIB_SpeedLoop_SF/6 -> pOutIQReq/1
  AMCLIB_SpeedLoop_SF/5 -> Delay17/1

== system ammclib_bam_s32k11x/AMCLIB/bam_f16/AMCLIB_TrackObsrv_F16 ==
  note: ---------------------------------------------------------------------------------------------------------------------------------------------------------------------------------------------------
  f16PhaseErr : Inport
  f16UpperLimit : Inport  Port=2
  f16LowerLimit : Inport  Port=3
  AMCLIB_TrackObsrv_SF : S-Function  FunctionName=AMCLIB_TrackObsrv_SF_F16  Parameters=f16CC1sc,f16CC2sc,u16NShift,f16C1,u16IntegNShift  SFunctionDeploymentMode=off  EnableBusSupport=off
  Unit_Delay_f16InErrK1 : Delay  DelayLength=1  InitialCondition=0
  Unit_Delay_f16InK1 : Delay  DelayLength=1  InitialCondition=0
  Unit_Delay_f32Acc : Delay  DelayLength=1  InitialCondition=0
  Unit_Delay_f32State : Delay  DelayLength=1  InitialCondition=0
  copyright : Subsystem
      mask Display: text(10,90,'FILE:');text(10,75,'DESRIPTION:');text(10,60,'COPYRIGHT:');text(10,45,'VERSION:');text(10,30,'DATE:')
  copyright2 : Subsystem
      mask Display: text(10,90,'AMCLIB_TrackObsrv_BAM_F16.mdl');text(10,75,'Tracking observer function.');text(10,60,'NXP');text(10,45,'1.0');text(10,30,'29-Jul-2016');
  logo : Subsystem
      mask Display: image(imread('logo.jpg'))
  f16PosEst : Outport
  f16VelocityEst : Outport  Port=2
  wires:
  AMCLIB_TrackObsrv_SF/2 -> f16VelocityEst/1
  AMCLIB_TrackObsrv_SF/1 -> f16PosEst/1
  f16LowerLimit/1 -> AMCLIB_TrackObsrv_SF/5
  f16UpperLimit/1 -> AMCLIB_TrackObsrv_SF/4
  f16PhaseErr/1 -> AMCLIB_TrackObsrv_SF/1
  Unit_Delay_f16InK1/1 -> AMCLIB_TrackObsrv_SF/7
  Unit_Delay_f32State/1 -> AMCLIB_TrackObsrv_SF/6
  Unit_Delay_f16InErrK1/1 -> AMCLIB_TrackObsrv_SF/3
  Unit_Delay_f32Acc/1 -> AMCLIB_TrackObsrv_SF/2
  AMCLIB_TrackObsrv_SF/6 -> Unit_Delay_f16InK1/1
  AMCLIB_TrackObsrv_SF/5 -> Unit_Delay_f32State/1
  AMCLIB_TrackObsrv_SF/4 -> Unit_Delay_f16InErrK1/1
  AMCLIB_TrackObsrv_SF/3 -> Unit_Delay_f32Acc/1

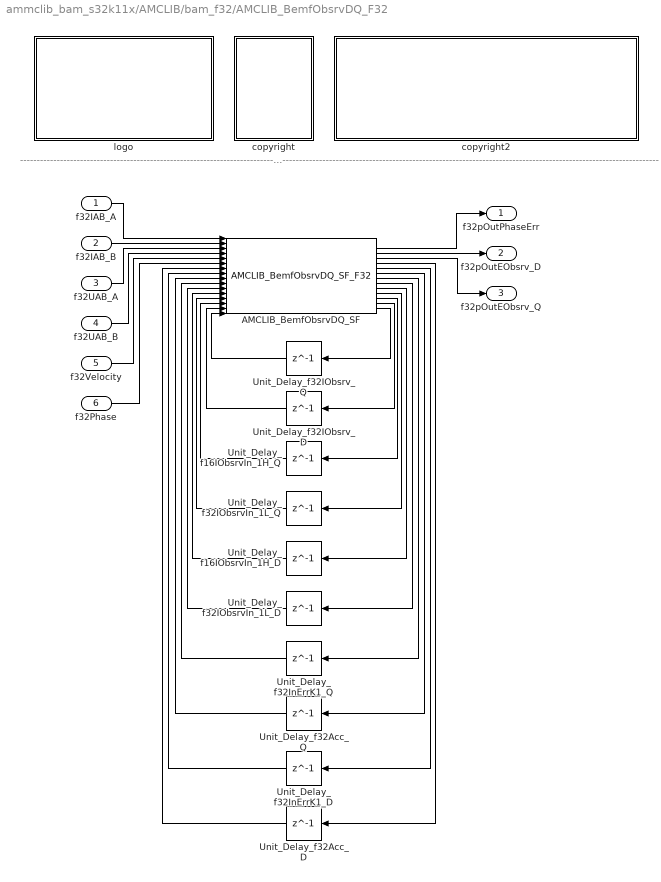
== system ammclib_bam_s32k11x/AMCLIB/bam_f32/AMCLIB_BemfObsrvDQ_F32 ==
  note: ---------------------------------------------------------------------------------------------------------------------------------------------------------------------------------------------------
  f32IAB_A : Inport
  f32IAB_B : Inport  Port=2
  f32UAB_A : Inport  Port=3
  f32UAB_B : Inport  Port=4
  f32Velocity : Inport  Port=5
  f32Phase : Inport  Port=6
  AMCLIB_BemfObsrvDQ_SF : S-Function  FunctionName=AMCLIB_BemfObsrvDQ_SF_F32  Parameters=f32IGain,f32UGain,f32WIGain,f32EGain,s16Shift,f32CC1sc_D,f32CC1sc_Q,f32CC2sc_D,f32CC2sc_Q,f32UpperLimit_D,f32UpperLimit_Q,f32LowerLimit_D,f32LowerLimit_Q,u16NShift  SFunctionDeploymentMode=off  EnableBusSupport=off
  Unit_Delay_f16IObsrvIn_1H_D : Delay  DelayLength=1  InitialCondition=0
  Unit_Delay_f16IObsrvIn_1H_Q : Delay  DelayLength=1  InitialCondition=0
  Unit_Delay_f32Acc_D : Delay  DelayLength=1  InitialCondition=0
  Unit_Delay_f32Acc_Q : Delay  DelayLength=1  InitialCondition=0
  Unit_Delay_f32IObsrvIn_1L_D : Delay  DelayLength=1  InitialCondition=0
  Unit_Delay_f32IObsrvIn_1L_Q : Delay  DelayLength=1  InitialCondition=0
  Unit_Delay_f32IObsrv_D : Delay  DelayLength=1  InitialCondition=0
  Unit_Delay_f32IObsrv_Q : Delay  DelayLength=1  InitialCondition=0
  Unit_Delay_f32InErrK1_D : Delay  DelayLength=1  InitialCondition=0
  Unit_Delay_f32InErrK1_Q : Delay  DelayLength=1  InitialCondition=0
  copyright : Subsystem
      mask Display: text(10,90,'FILE:');text(10,75,'DESRIPTION:');text(10,60,'COPYRIGHT:');text(10,45,'VERSION:');text(10,30,'DATE:')
  copyright2 : Subsystem
      mask Display: text(10,90,'AMCLIB_BemfObsrvDQ_BAM_F32.mdl');text(10,75,'PMSM back-EMF observer DQ.');text(10,60,'NXP');text(10,45,'1.0');text(10,30,'26-Oct-2016');
  logo : Subsystem
      mask Display: image(imread('logo.jpg'))
  f32pOutPhaseErr : Outport
  f32pOutEObsrv_D : Outport  Port=2
  f32pOutEObsrv_Q : Outport  Port=3
  wires:
  AMCLIB_BemfObsrvDQ_SF/3 -> f32pOutEObsrv_Q/1
  AMCLIB_BemfObsrvDQ_SF/2 -> f32pOutEObsrv_D/1
  AMCLIB_BemfObsrvDQ_SF/1 -> f32pOutPhaseErr/1
  f32Phase/1 -> AMCLIB_BemfObsrvDQ_SF/6
  f32Velocity/1 -> AMCLIB_BemfObsrvDQ_SF/5
  f32UAB_B/1 -> AMCLIB_BemfObsrvDQ_SF/4
  f32UAB_A/1 -> AMCLIB_BemfObsrvDQ_SF/3
  f32IAB_B/1 -> AMCLIB_BemfObsrvDQ_SF/2
  f32IAB_A/1 -> AMCLIB_BemfObsrvDQ_SF/1
  Unit_Delay_f32IObsrv_Q/1 -> AMCLIB_BemfObsrvDQ_SF/16
  Unit_Delay_f32IObsrv_D/1 -> AMCLIB_BemfObsrvDQ_SF/15
  Unit_Delay_f16IObsrvIn_1H_Q/1 -> AMCLIB_BemfObsrvDQ_SF/14
  AMCLIB_BemfObsrvDQ_SF/13 -> Unit_Delay_f32IObsrv_Q/1
  AMCLIB_BemfObsrvDQ_SF/12 -> Unit_Delay_f32IObsrv_D/1
  AMCLIB_BemfObsrvDQ_SF/11 -> Unit_Delay_f16IObsrvIn_1H_Q/1
  AMCLIB_BemfObsrvDQ_SF/10 -> Unit_Delay_f32IObsrvIn_1L_Q/1
  Unit_Delay_f32IObsrvIn_1L_Q/1 -> AMCLIB_BemfObsrvDQ_SF/13
  Unit_Delay_f16IObsrvIn_1H_D/1 -> AMCLIB_BemfObsrvDQ_SF/12
  AMCLIB_BemfObsrvDQ_SF/9 -> Unit_Delay_f16IObsrvIn_1H_D/1
  AMCLIB_BemfObsrvDQ_SF/8 -> Unit_Delay_f32IObsrvIn_1L_D/1
  Unit_Delay_f32IObsrvIn_1L_D/1 -> AMCLIB_BemfObsrvDQ_SF/11
  Unit_Delay_f32InErrK1_Q/1 -> AMCLIB_BemfObsrvDQ_SF/10
  AMCLIB_BemfObsrvDQ_SF/7 -> Unit_Delay_f32InErrK1_Q/1
  AMCLIB_BemfObsrvDQ_SF/6 -> Unit_Delay_f32Acc_Q/1
  Unit_Delay_f32Acc_Q/1 -> AMCLIB_BemfObsrvDQ_SF/9
  Unit_Delay_f32InErrK1_D/1 -> AMCLIB_BemfObsrvDQ_SF/8
  Unit_Delay_f32Acc_D/1 -> AMCLIB_BemfObsrvDQ_SF/7
  AMCLIB_BemfObsrvDQ_SF/5 -> Unit_Delay_f32InErrK1_D/1
  AMCLIB_BemfObsrvDQ_SF/4 -> Unit_Delay_f32Acc_D/1

== system ammclib_bam_s32k11x/AMCLIB/bam_f32/AMCLIB_CurrentLoop_F32 ==
  note: ---------------------------------------------------------------------------------------------------------------------------------------------------------------------------------------------------
  f32UDcBus : Inport
  f32IDReq : Inport  Port=2
  f32IQReq : Inport  Port=3
  f32IDFbck : Inport  Port=4
  f32IQFbck : Inport  Port=5
  AMCLIB_CurrentLoop_SF : S-Function  FunctionName=AMCLIB_CurrentLoop_SF_F32  Parameters=f32CC1scD,f32CC2scD,u16NShiftD,f32CC1scQ,f32CC2scQ,u16NShiftQ  SFunctionDeploymentMode=off  EnableBusSupport=off
  Delay{30..33} (4 alike) : Delay  DelayLength=1  InitialCondition=0
  copyright : Subsystem
      mask Display: text(10,90,'FILE:');text(10,75,'DESRIPTION:');text(10,60,'COPYRIGHT:');text(10,45,'VERSION:');text(10,30,'DATE:')
  copyright2 : Subsystem
      mask Display: text(10,90,'AMCLIB_CurrentLoop_BAM_F32.mdl');text(10,75,'PMSM Current Loop.');text(10,60,'NXP');text(10,45,'1.0');text(10,30,'25-Oct-2017');
  logo : Subsystem
      mask Display: image(imread('logo.jpg'))
  pOutUDReq : Outport
  pOutUQReq : Outport  Port=2
  wires:
  f32UDcBus/1 -> AMCLIB_CurrentLoop_SF/1
  f32IDReq/1 -> AMCLIB_CurrentLoop_SF/2
  f32IQReq/1 -> AMCLIB_CurrentLoop_SF/3
  f32IDFbck/1 -> AMCLIB_CurrentLoop_SF/4
  f32IQFbck/1 -> AMCLIB_CurrentLoop_SF/5
  Delay32/1 -> AMCLIB_CurrentLoop_SF/6
  Delay31/1 -> AMCLIB_CurrentLoop_SF/7
  Delay30/1 -> AMCLIB_CurrentLoop_SF/8
  Delay33/1 -> AMCLIB_CurrentLoop_SF/9
  AMCLIB_CurrentLoop_SF/1 -> Delay32/1
  AMCLIB_CurrentLoop_SF/2 -> Delay31/1
  AMCLIB_CurrentLoop_SF/3 -> Delay30/1
  AMCLIB_CurrentLoop_SF/4 -> Delay33/1
  AMCLIB_CurrentLoop_SF/5 -> pOutUDReq/1
  AMCLIB_CurrentLoop_SF/6 -> pOutUQReq/1

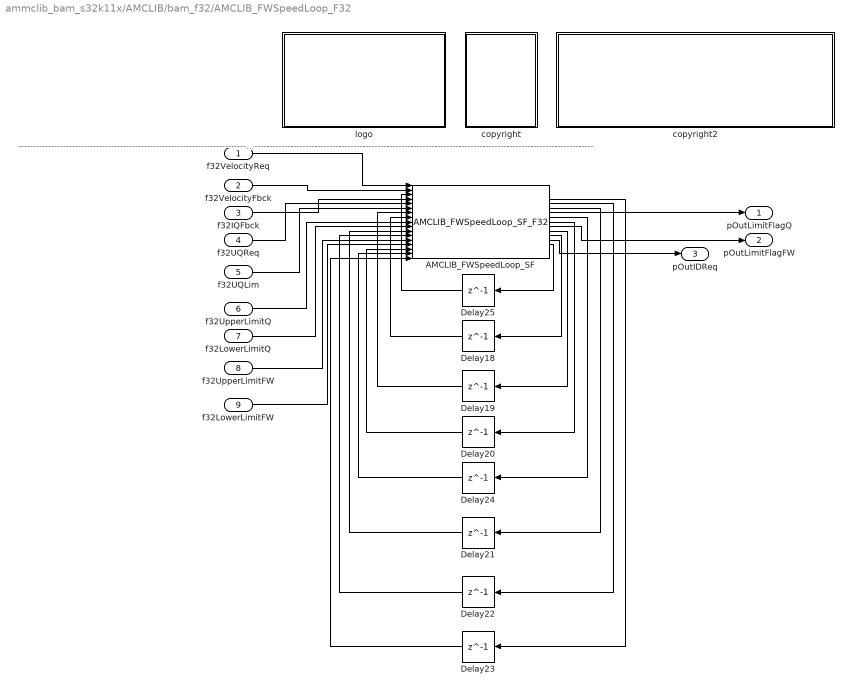
== system ammclib_bam_s32k11x/AMCLIB/bam_f32/AMCLIB_FWSpeedLoop_F32 ==
  note: ---------------------------------------------------------------------------------------------------------------------------------------------------------------------------------------------------
  f32VelocityReq : Inport
  f32VelocityFbck : Inport  Port=2
  f32IQFbck : Inport  Port=3
  f32UQReq : Inport  Port=4
  f32UQLim : Inport  Port=5
  f32UpperLimitQ : Inport  Port=6
  f32LowerLimitQ : Inport  Port=7
  f32UpperLimitFW : Inport  Port=8
  f32LowerLimitFW : Inport  Port=9
  AMCLIB_FWSpeedLoop_SF : S-Function  FunctionName=AMCLIB_FWSpeedLoop_SF_F32  Parameters=u16NSamplesW,u16NSamplesFW,f32PropGainQ,s16PropGainShiftQ,f32IntegGainQ,s16IntegGainShiftQ,f32PropGainFW,s16PropGainShiftFW,f32IntegGainFW,s16IntegGainShiftFW,f32RampUp,f32RampDown  SFunctionDeploymentMode=off  EnableBusSupport=off
  Delay{18..25} (8 alike) : Delay  DelayLength=1  InitialCondition=0
  copyright : Subsystem
      mask Display: text(10,90,'FILE:');text(10,75,'DESRIPTION:');text(10,60,'COPYRIGHT:');text(10,45,'VERSION:');text(10,30,'DATE:')
  copyright2 : Subsystem
      mask Display: text(10,90,'AMCLIB_FWSpeedLoop_BAM_F32.mdl');text(10,75,'Speed Loop with Field Weakening.');text(10,60,'NXP');text(10,45,'1.0');text(10,30,'28-Aug-2017');
  logo : Subsystem
      mask Display: image(imread('logo.jpg'))
  pOutLimitFlagQ : Outport
  pOutLimitFlagFW : Outport  Port=2
  pOutIDReq : Outport  Port=3
  wires:
  f32VelocityReq/1 -> AMCLIB_FWSpeedLoop_SF/1
  f32VelocityFbck/1 -> AMCLIB_FWSpeedLoop_SF/2
  Delay25/1 -> AMCLIB_FWSpeedLoop_SF/3
  f32IQFbck/1 -> AMCLIB_FWSpeedLoop_SF/4
  f32UQReq/1 -> AMCLIB_FWSpeedLoop_SF/5
  f32UQLim/1 -> AMCLIB_FWSpeedLoop_SF/6
  Delay19/1 -> AMCLIB_FWSpeedLoop_SF/7
  Delay18/1 -> AMCLIB_FWSpeedLoop_SF/8
  f32UpperLimitQ/1 -> AMCLIB_FWSpeedLoop_SF/9
  f32LowerLimitQ/1 -> AMCLIB_FWSpeedLoop_SF/10
  Delay21/1 -> AMCLIB_FWSpeedLoop_SF/11
  Delay22/1 -> AMCLIB_FWSpeedLoop_SF/12
  f32UpperLimitFW/1 -> AMCLIB_FWSpeedLoop_SF/13
  f32LowerLimitFW/1 -> AMCLIB_FWSpeedLoop_SF/14
  Delay20/1 -> AMCLIB_FWSpeedLoop_SF/15
  Delay24/1 -> AMCLIB_FWSpeedLoop_SF/16
  Delay23/1 -> AMCLIB_FWSpeedLoop_SF/17
  AMCLIB_FWSpeedLoop_SF/1 -> Delay23/1
  AMCLIB_FWSpeedLoop_SF/2 -> Delay22/1
  AMCLIB_FWSpeedLoop_SF/3 -> Delay21/1
  AMCLIB_FWSpeedLoop_SF/4 -> pOutLimitFlagQ/1
  AMCLIB_FWSpeedLoop_SF/5 -> Delay24/1
  AMCLIB_FWSpeedLoop_SF/6 -> Delay20/1
  AMCLIB_FWSpeedLoop_SF/7 -> pOutLimitFlagFW/1
  AMCLIB_FWSpeedLoop_SF/8 -> Delay19/1
  AMCLIB_FWSpeedLoop_SF/9 -> Delay18/1
  AMCLIB_FWSpeedLoop_SF/10 -> pOutIDReq/1
  AMCLIB_FWSpeedLoop_SF/11 -> Delay25/1

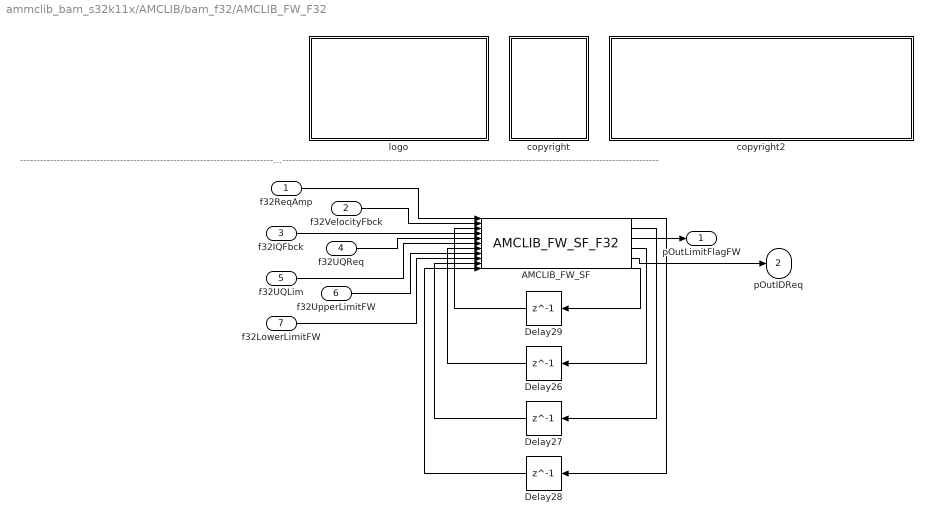
== system ammclib_bam_s32k11x/AMCLIB/bam_f32/AMCLIB_FW_F32 ==
  note: ---------------------------------------------------------------------------------------------------------------------------------------------------------------------------------------------------
  f32ReqAmp : Inport
  f32VelocityFbck : Inport  Port=2
  f32IQFbck : Inport  Port=3
  f32UQReq : Inport  Port=4
  f32UQLim : Inport  Port=5
  f32UpperLimitFW : Inport  Port=6
  f32LowerLimitFW : Inport  Port=7
  AMCLIB_FW_SF : S-Function  FunctionName=AMCLIB_FW_SF_F32  Parameters=u16NSamplesFW,f32PropGainFW,s16PropGainShiftFW,f32IntegGainFW,s16IntegGainShiftFW  SFunctionDeploymentMode=off  EnableBusSupport=off
  Delay{26..29} (4 alike) : Delay  DelayLength=1  InitialCondition=0
  copyright : Subsystem
      mask Display: text(10,90,'FILE:');text(10,75,'DESRIPTION:');text(10,60,'COPYRIGHT:');text(10,45,'VERSION:');text(10,30,'DATE:')
  copyright2 : Subsystem
      mask Display: text(10,90,'AMCLIB_FW_BAM_F32.mdl');text(10,75,'Speed Loop with Field Weakening.');text(10,60,'NXP');text(10,45,'1.0');text(10,30,'28-Aug-2017');
  logo : Subsystem
      mask Display: image(imread('logo.jpg'))
  pOutLimitFlagFW : Outport
  pOutIDReq : Outport  Port=2
  wires:
  f32ReqAmp/1 -> AMCLIB_FW_SF/1
  f32VelocityFbck/1 -> AMCLIB_FW_SF/2
  Delay29/1 -> AMCLIB_FW_SF/3
  f32IQFbck/1 -> AMCLIB_FW_SF/4
  f32UQReq/1 -> AMCLIB_FW_SF/5
  f32UQLim/1 -> AMCLIB_FW_SF/6
  Delay26/1 -> AMCLIB_FW_SF/7
  f32UpperLimitFW/1 -> AMCLIB_FW_SF/8
  f32LowerLimitFW/1 -> AMCLIB_FW_SF/9
  Delay27/1 -> AMCLIB_FW_SF/10
  Delay28/1 -> AMCLIB_FW_SF/11
  AMCLIB_FW_SF/1 -> Delay28/1
  AMCLIB_FW_SF/2 -> Delay27/1
  AMCLIB_FW_SF/3 -> pOutLimitFlagFW/1
  AMCLIB_FW_SF/4 -> Delay26/1
  AMCLIB_FW_SF/5 -> pOutIDReq/1
  AMCLIB_FW_SF/6 -> Delay29/1

== system ammclib_bam_s32k11x/AMCLIB/bam_f32/AMCLIB_SpeedLoop_F32 ==
  note: ---------------------------------------------------------------------------------------------------------------------------------------------------------------------------------------------------
  f32VelocityReq : Inport
  f32VelocityFbck : Inport  Port=2
  f32UpperLimitQ : Inport  Port=3
  f32LowerLimitQ : Inport  Port=4
  AMCLIB_SpeedLoop_SF : S-Function  FunctionName=AMCLIB_SpeedLoop_SF_F32  Parameters=u16NSamplesW,f32PropGainQ,s16PropGainShiftQ,f32IntegGainQ,s16IntegGainShiftQ,f32RampUp,f32RampDown  SFunctionDeploymentMode=off  EnableBusSupport=off
  Delay{1,14..15,17} (4 alike) : Delay  DelayLength=1  InitialCondition=0
  copyright : Subsystem
      mask Display: text(10,90,'FILE:');text(10,75,'DESRIPTION:');text(10,60,'COPYRIGHT:');text(10,45,'VERSION:');text(10,30,'DATE:')
  copyright2 : Subsystem
      mask Display: text(10,90,'AMCLIB_SpeedLoop_BAM_F32.mdl');text(10,75,'Speed Loop with Field Weakening.');text(10,60,'NXP');text(10,45,'1.0');text(10,30,'28-Aug-2017');
  logo : Subsystem
      mask Display: image(imread('logo.jpg'))
  pOutLimitFlagQ : Outport
  pOutIQReq : Outport  Port=2
  wires:
  f32VelocityReq/1 -> AMCLIB_SpeedLoop_SF/1
  f32VelocityFbck/1 -> AMCLIB_SpeedLoop_SF/2
  Delay17/1 -> AMCLIB_SpeedLoop_SF/3
  f32UpperLimitQ/1 -> AMCLIB_SpeedLoop_SF/4
  f32LowerLimitQ/1 -> AMCLIB_SpeedLoop_SF/5
  Delay14/1 -> AMCLIB_SpeedLoop_SF/6
  Delay15/1 -> AMCLIB_SpeedLoop_SF/7
  Delay1/1 -> AMCLIB_SpeedLoop_SF/8
  AMCLIB_SpeedLoop_SF/1 -> Delay1/1
  AMCLIB_SpeedLoop_SF/2 -> Delay15/1
  AMCLIB_SpeedLoop_SF/3 -> Delay14/1
  AMCLIB_SpeedLoop_SF/4 -> pOutLimitFlagQ/1
  AMCLIB_SpeedLoop_SF/5 -> Delay17/1
  AMCLIB_SpeedLoop_SF/6 -> pOutIQReq/1
